simulink model "fig1"  (R2016b)
settings: Solver=VariableStepAuto  StartTime=0.0  StopTime=10.0  RelTol=1e-3
values from neighbouring files (symbols this model uses):
  K = K_array(i)    [Lab2.m]    (also in lab2.m)
settings Model: Creator=ee105-abq  LastModifiedBy=ee105-abq

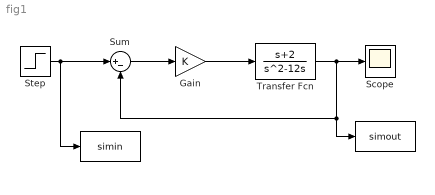
== system fig1 ==
  " " : ToWorkspace  VariableName=simout  SaveFormat=Timeseries  SampleTime=-1
  "  " : ToWorkspace  VariableName=simin  SaveFormat=Timeseries  SampleTime=-1
  Gain : Gain  Gain=K
  Scope : Scope
  Step : Step  SampleTime=0
  Sum : Sum  Inputs=|+-
  Transfer Fcn : TransferFcn  Numerator=[1 2]  Denominator=[1 -12 0]
  wires:
  Step/1 -> "  "/1, Sum/1
  Sum/1 -> Gain/1
  Gain/1 -> Transfer Fcn/1
  Transfer Fcn/1 -> Sum/2, " "/1, Scope/1
